simulink model "fixed_2"  (Simulink 7.8)
settings: Solver=FixedStepDiscrete  StartTime=0.0  StopTime=0.05  RelTol=1e-3
libraries: dspsigops x2, dspobslib x1
settings Model: Creator=svenhoffmann  LastModifiedBy=josef  ExtModeAutoUpdateStatusClock=off
settings OptimizationCC: InitFltsAndDblsToZero=on
settings DebuggingCC: SaveWithParameterizedLinksMsg=none  SignalResolutionControl=TryResolveAllWithWarning  MultiTaskDSMMsg=warning  MultiTaskCondExecSysMsg=none  FcnCallInpInsideContextMsg=Use local settings  StrictBusMsg=None
settings RTWCC: IncludeERTFirstTime=on
settings GRTTargetCC: TargetFcnLib=ansi_tfl_tmw.mat

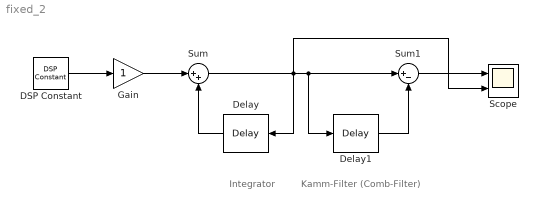
== system fixed_2 ==
  note: Integrator
  note: Kamm-Filter (Comb-Filter)
  DSP Constant : dspobslib/DSP Constant  Value=1  SampleMode=Discrete  discreteOutput=Sample-based  continuousOutput=Sample-based  sampTime=1/1000  framePeriod=2  dataType=User-defined  isSigned=on  wordLen=16  udDataType=sfix(2)  fracBitsMode=User-defined  numFracBits=0  InterpretAs1D=-inf  Ts=-inf  FramebasedOutput=-inf
  Delay : dspsigops/Delay  InputProcessing=Inherited (this choice will be removed - see release notes)  dly_unit=Samples  delay=1  ic_detail=off  dif_ic_for_ch=off  dif_ic_for_dly=off  ic=0  reset_popup=None
  Delay1 : dspsigops/Delay  InputProcessing=Inherited (this choice will be removed - see release notes)  dly_unit=Samples  delay=4  ic_detail=off  dif_ic_for_ch=off  dif_ic_for_dly=off  ic=0  reset_popup=None
  Gain : Gain  ParamDataTypeStr=fixdt(1,16,12)  OutDataTypeStr=fixdt(1,4,0)  SaturateOnIntegerOverflow=on
  Scope : Scope  NumInputPorts=2
      settings: YMin=0~-5  YMax=5~5
  Sum : Sum  Inputs=|++  OutDataTypeStr=Inherit: Inherit via back propagation
  Sum1 : Sum  Inputs=|+-  OutDataTypeStr=Inherit: Inherit via back propagation
  wires:
  DSP Constant/1 -> Gain/1
  Gain/1 -> Sum/1
  Delay/1 -> Sum/2
  Sum/1 -> Sum1/1, Delay1/1, Scope/2, Delay/1
  Delay1/1 -> Sum1/2
  Sum1/1 -> Scope/1
